simulink model "twolink_PD"  (R2017b)
settings: Solver=VariableStepAuto  StartTime=0.0  StopTime=20  RelTol=1e-3
values from neighbouring files (symbols this model uses):
  h = diff(x)    [dfdx.m]    (also in inv_control.m = -m2*l1*lc2*sin(q2); twolink_ftraj.m = 0.1; twolink_valid.m = 0.1)
libraries: roblocks x1
settings Model: Creator=sathish  LastModifiedBy=sathish

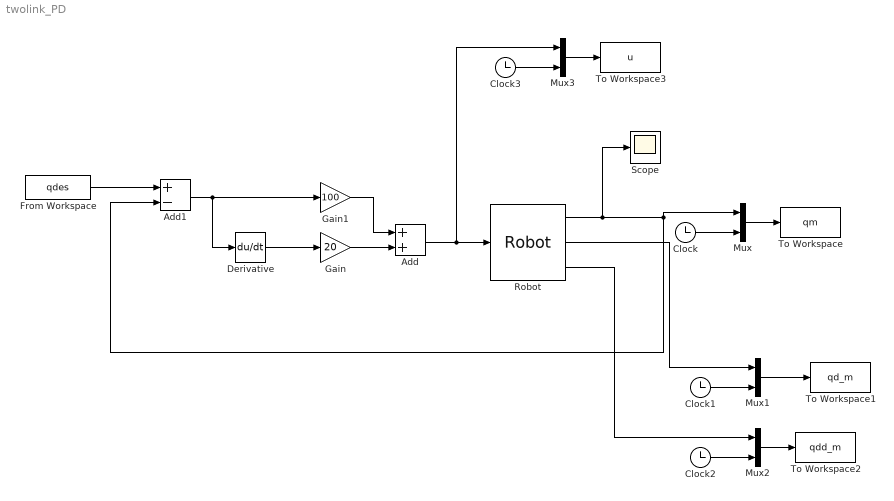
== system twolink_PD ==
  Add : Sum
  Add1 : Sum  Inputs=+-
  Clock{,1..3} (4 alike) : Clock
  Derivative : Derivative
  From Workspace : FromWorkspace  VariableName=qdes  SampleTime=h
  Gain : Gain  Gain=20
  Gain1 : Gain  Gain=100
  Mux{,1..3} (4 alike) : Mux  Inputs=2
  Robot : roblocks/Arm/Robot  robot=twolink_mod  q0=[0 0]
  Scope : Scope
  To Workspace : ToWorkspace  VariableName=qm  SaveFormat=Timeseries  SampleTime=h
  To Workspace1 : ToWorkspace  VariableName=qd_m  SaveFormat=Timeseries  SampleTime=h
  To Workspace2 : ToWorkspace  VariableName=qdd_m  SaveFormat=Timeseries  SampleTime=h
  To Workspace3 : ToWorkspace  VariableName=u  SaveFormat=Timeseries  SampleTime=h
  wires:
  Robot/1 -> Mux/1, Add1/2, Scope/1
  Clock/1 -> Mux/2
  From Workspace/1 -> Add1/1
  Mux/1 -> To Workspace/1
  Add1/1 -> Gain1/1, Derivative/1
  Derivative/1 -> Gain/1
  Gain/1 -> Add/2
  Gain1/1 -> Add/1
  Robot/2 -> Mux1/1
  Mux1/1 -> To Workspace1/1
  Clock1/1 -> Mux1/2
  Robot/3 -> Mux2/1
  Mux2/1 -> To Workspace2/1
  Clock2/1 -> Mux2/2
  Add/1 -> Mux3/1, Robot/1
  Mux3/1 -> To Workspace3/1
  Clock3/1 -> Mux3/2
